simulink model "rtwdemo_structsignal"  (Simulink 7.1)
settings: Solver=FixedStepDiscrete  StartTime=0.0  StopTime=10.0  RelTol=1e-3
PostLoadFcn:
  | load structsignal.mat;
settings Model: Creator=ajayaram  LastModifiedBy=ajayaram
settings OptimizationCC: InlineParams=on  OptimizeModelRefInitCode=on  LifeSpan=1
settings RTWCC: SystemTargetFile=ert.tlc  GenCodeOnly=on  GenerateMakefile=off  TemplateMakefile=ert_default_tmf  Description=Real-Time Workshop Embedded Coder (no auto configuration)  GenerateReport=on  ProcessScript=ert_make_rtw_hook  IncludeHyperlinkInReport=on  LaunchReport=on
settings CodeAppCC: IgnoreCustomStorageClasses=off
settings ERTTargetCC: GenerateSampleERTMain=on  InlinedParameterPlacement=NonHierarchical  ERTCustomFileTemplate=example_file_process.tlc

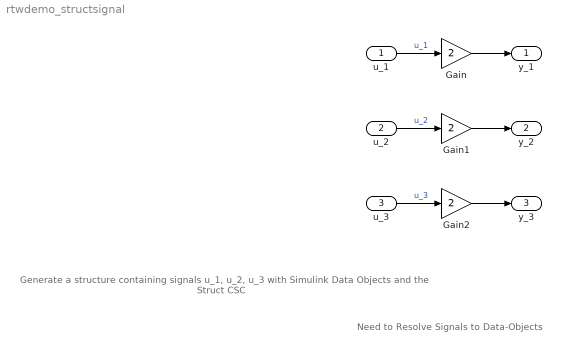
== system rtwdemo_structsignal ==
  note: Need to Resolve Signals to Data-Objects
  note: Generate a structure containing signals
      | u_1, u_2, u_3 with Simulink Data Objects and the Struct CSC
  u_1 : Inport  OutDataType=sfix(16)  OutScaling=2^0
  u_2 : Inport  Port=2  OutDataType=sfix(16)  OutScaling=2^0
  u_3 : Inport  Port=3  OutDataType=sfix(16)  OutScaling=2^0
  Gain : Gain  Gain=2  ParameterDataType=sfix(16)  ParameterScaling=2^0  OutDataType=sfix(16)  OutScaling=2^0
  Gain1 : Gain  Gain=2  ParameterDataType=sfix(16)  ParameterScaling=2^0  OutDataType=sfix(16)  OutScaling=2^0
  Gain2 : Gain  Gain=2  ParameterDataType=sfix(16)  ParameterScaling=2^0  OutDataType=sfix(16)  OutScaling=2^0
  y_1 : Outport  OutDataType=sfix(16)  OutScaling=2^0
  y_2 : Outport  Port=2  OutDataType=sfix(16)  OutScaling=2^0
  y_3 : Outport  Port=3  OutDataType=sfix(16)  OutScaling=2^0
  wires:
  u_1/1 -> Gain/1  "u_1"
  u_2/1 -> Gain1/1  "u_2"
  u_3/1 -> Gain2/1  "u_3"
  Gain/1 -> y_1/1
  Gain1/1 -> y_2/1
  Gain2/1 -> y_3/1
